simulink subsystem "PvtSubSys_VSM_LKA"  (R2020b)
settings: Solver=VariableStepAuto  StartTime=0.0  StopTime=10.0  RelTol=1e-3
values from neighbouring files (symbols this model uses):
  P_VSM_LKA_AbsEspInTime = 3.0    [LKA.sldd]
  P_VSM_LKA_absLongitudeAcceIn = 2.5    [LKA.sldd]
  P_VSM_LKA_absLongitudeAcceInTime = 3.0    [LKA.sldd]
  P_VSM_LKA_absLongitudeAcceOut = 3.0    [LKA.sldd]
  P_VSM_LKA_AccPedalPosnOut = 30.0    [LKA.sldd]
  P_VSM_LKA_AccPedalRateOutTime = 0.0    [LKA.sldd]
  P_VSM_LKA_AccRateIn = 30.0    [LKA.sldd]
  P_VSM_LKA_AccRateInTime = 1.5    [LKA.sldd]
  P_VSM_LKA_AccRateOut = 70.0    [LKA.sldd]
  P_VSM_LKA_BrakePressIn = 3.0    [LKA.sldd]
  P_VSM_LKA_BrakePressInTime = 1.5    [LKA.sldd]
  P_VSM_LKA_BrakePressOut = 5.0    [LKA.sldd]
  P_VSM_LKA_CurveFactor = 1.0    [LKA.sldd]
  P_VSM_LKA_DriverInputTrqValueIn = 2.0    [LKA.sldd]
  P_VSM_LKA_DriverInputTrqValueInTime = 3.0    [LKA.sldd]
  P_VSM_LKA_DriverInputTrqValueOut = 2.3    [LKA.sldd]
  P_VSM_LKA_EndSwitch = 1.0    [LKA.sldd]
  P_VSM_LKA_LaneChangeOffset = 0.11    [LKA.sldd]
  P_VSM_LKA_LaneCurveIn = 0.005    [LKA.sldd]
  P_VSM_LKA_LaneCurveOut = 0.006    [LKA.sldd]
  P_VSM_LKA_LateralAcceIn = 3.0    [LKA.sldd]
  P_VSM_LKA_LateralAcceInTime = 3.0    [LKA.sldd]
  P_VSM_LKA_LateralAcceOut = 3.5    [LKA.sldd]
  P_VSM_LKA_LongitudeAcceIn = 3.0    [LKA.sldd]
  P_VSM_LKA_LongitudeAcceOut = 3.5    [LKA.sldd]
  P_VSM_LKA_OverrideInTime = 1.5    [LKA.sldd]
  P_VSM_LKA_OverrideTime = 0.3    [LKA.sldd]
  P_VSM_LKA_OverrideValue = 1.2    [LKA.sldd]
  P_VSM_LKA_State_Absesp_enable = 1.0    [LKA.sldd]
  P_VSM_LKA_State_Accpedalrate_enable = 1.0    [LKA.sldd]
  P_VSM_LKA_State_Breakpressure_enable = 1.0    [LKA.sldd]
  P_VSM_LKA_State_DriverInputTrqValue_enable = 1.0    [LKA.sldd]
  P_VSM_LKA_State_Eps_enable = 1.0    [LKA.sldd]
  P_VSM_LKA_State_ESSSts_enable = 1.0    [LKA.sldd]
  P_VSM_LKA_State_Failsafe_enable = 1.0    [LKA.sldd]
  P_VSM_LKA_State_GEAR_enable = 1.0    [LKA.sldd]
  P_VSM_LKA_State_Handson_enable = 1.0    [LKA.sldd]
  P_VSM_LKA_State_Headingangle_enable = 1.0    [LKA.sldd]
  P_VSM_LKA_State_Lane_enable = 1.0    [LKA.sldd]
  P_VSM_LKA_State_LaneChange_enable = 1.0    [LKA.sldd]
  P_VSM_LKA_State_Lanecurve_enable = 1.0    [LKA.sldd]
  P_VSM_LKA_State_LateralAcce_enable = 1.0    [LKA.sldd]
  P_VSM_LKA_State_LongitudeAcc_enable = 1.0    [LKA.sldd]
  P_VSM_LKA_State_Overide_enable = 1.0    [LKA.sldd]
  P_VSM_LKA_State_Param_AngleOffset = 0.15    [LKA.sldd]
  P_VSM_LKA_State_Param_InterventionZoneIn = 0.4    [LKA.sldd]
  P_VSM_LKA_State_Param_InterventionZoneOut = -0.65    [LKA.sldd]
  P_VSM_LKA_State_Param_LaneCurve : value not decoded    [LKA.sldd]
  P_VSM_LKA_State_Param_LaneCurve_Offset : value not decoded    [LKA.sldd]
  P_VSM_LKA_State_Param_LaneWidth_Offset : value not decoded    [LKA.sldd]
  P_VSM_LKA_State_Param_OutOffset = 0.2    [LKA.sldd]
  P_VSM_LKA_State_Param_REInterventionZoneIn = 0.55    [LKA.sldd]
  P_VSM_LKA_State_Param_Sensitive_Offset : value not decoded    [LKA.sldd]
  P_VSM_LKA_State_SteerWheelAngle_enable = 1.0    [LKA.sldd]
  P_VSM_LKA_State_SteerWheelSpd_enable = 1.0    [LKA.sldd]
  P_VSM_LKA_State_TJASts_enable = 1.0    [LKA.sldd]
  P_VSM_LKA_State_TurnLight_enable = 1.0    [LKA.sldd]
  P_VSM_LKA_State_Vehspeed_enable = 1.0    [LKA.sldd]
  P_VSM_LKA_State_Yawsup_enable = 1.0    [LKA.sldd]
  P_VSM_LKA_SteerWheelAngleIn = 70.0    [LKA.sldd]
  P_VSM_LKA_SteerWheelAngleInTime = 3.0    [LKA.sldd]
  P_VSM_LKA_SteerWheelAngleOut = 90.0    [LKA.sldd]
  P_VSM_LKA_SteerWheelSpdIn = 150.0    [LKA.sldd]
  P_VSM_LKA_SteerWheelSpdInTime = 3.0    [LKA.sldd]
  P_VSM_LKA_SteerWheelSpdOut = 200.0    [LKA.sldd]
  P_VSM_LKA_TurnLightInTime = 3.0    [LKA.sldd]
  P_VSM_LKA_Warnarea1 = -0.55    [LKA.sldd]
  P_VSM_LKA_Warnarea2 = -0.35    [LKA.sldd]
  P_VSM_LKA_WarnInTime = 2.0    [LKA.sldd]
  P_VSM_LKA_WhelDy = 2.0    [LKA.sldd]
  P_VSM_LKA_YawRateIn = 0.2    [LKA.sldd]
  P_VSM_LKA_YawRateInTime = 1.0    [LKA.sldd]
  P_VSM_LKA_YawRateOut = 0.25    [LKA.sldd]
undefined symbols (not defined in the file or in its folder): P_VSM_LKA_AddOffset, P_VSM_LSMC_SampleTime, STATE
libraries: simulink x162
(part 2 of 5)

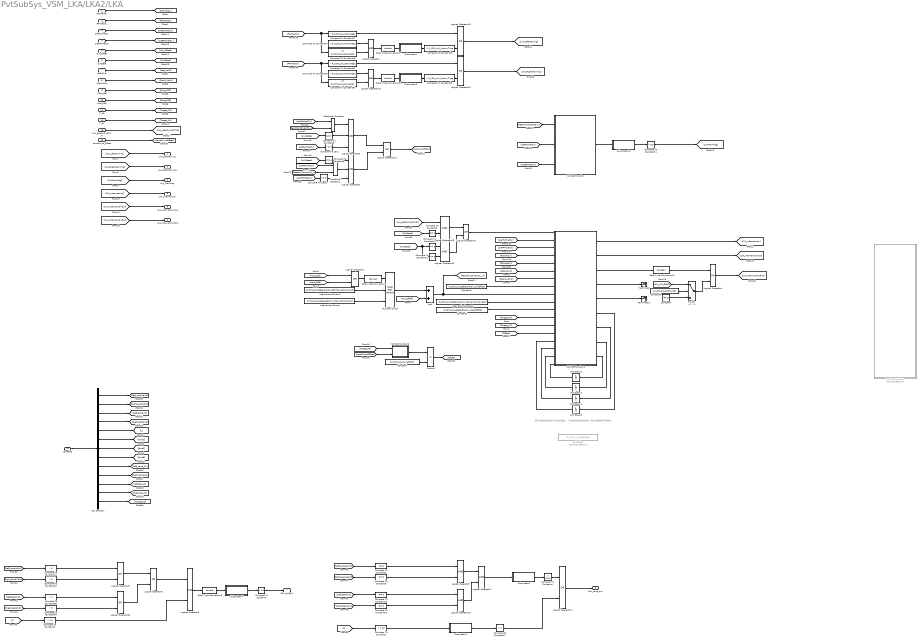
== system PvtSubSys_VSM_LKA/LKA2/LKA ==
  note: 基于车道线存在条件下成立的逻辑，一旦去掉车道线存在条件，那么该逻辑将不复存在；
  FLWhelDy : Inport
  FRWhelDy : Inport  Port=2
  preFLWhelDy : Inport  Port=3
  preFRWhelDy : Inport  Port=4
  LKA_Offset : Inport  Port=5
  LKAState : Inport  Port=6
  LeftValid : Inport  Port=7
  RightValid : Inport  Port=8
  Host_LRE : Inport  Port=9
  Host_RRE : Inport  Port=10
  T_A0 : Inport  Port=11
  T_A1 : Inport  Port=12
  LKA_READY2ACTIVE : Inport  Port=13
  LaneARe : Inport  Port=14
  LaneCurve_Offset : Inport  Port=15
  Add : Sum
  Bus Selector : BusSelector  OutputSignals=Left_LaneValid,Right_LaneValid,Left_ReValid,Right_ReValid,LDWLKAELK_LWidth,Signal_Lane1,Signal_Lane2,Signal_Lane3,Left_Lane_A1,Right_Lane_A1,Left_Re_A1,Right_Re_A1,T_A2
  Compare To Constant1 : simulink/Logic and Bit Operations/Compare To Constant  relop=<  const=2.45  OutDataTypeStr=boolean
  Compare To Constant10 : simulink/Logic and Bit Operations/Compare To Constant  relop=>=  const=3  OutDataTypeStr=boolean
  Compare To Constant11 : simulink/Logic and Bit Operations/Compare To Constant  relop=<=  const=5  OutDataTypeStr=boolean
  Compare To Constant12 : simulink/Logic and Bit Operations/Compare To Constant  relop=>  const=1  OutDataTypeStr=boolean
  Compare To Constant{3,6,13..14} (4 alike) : simulink/Logic and Bit Operations/Compare To Constant  relop===  const=0  OutDataTypeStr=boolean
  Compare To Constant{16,18,68,84} (4 alike) : simulink/Logic and Bit Operations/Compare To Constant  relop=>  const=0  OutDataTypeStr=boolean
  Compare To Constant2 : simulink/Logic and Bit Operations/Compare To Constant  relop=>  const=2.5  OutDataTypeStr=boolean
  Compare To Constant4 : simulink/Logic and Bit Operations/Compare To Constant  relop=>  const=0.25  OutDataTypeStr=boolean
  Compare To Constant44 : simulink/Logic and Bit Operations/Compare To Constant  relop=<  const=P_VSM_LKA_Warnarea2  OutDataTypeStr=boolean
  Compare To Constant45 : simulink/Logic and Bit Operations/Compare To Constant  relop=>  const=P_VSM_LKA_WarnInTime  OutDataTypeStr=boolean
  Compare To Constant46 : simulink/Logic and Bit Operations/Compare To Constant  relop=>=  const=P_VSM_LKA_Warnarea1  OutDataTypeStr=boolean
  Compare To Constant47 : simulink/Logic and Bit Operations/Compare To Constant  relop=<  const=P_VSM_LKA_Warnarea1  OutDataTypeStr=boolean
  Compare To Constant48 : simulink/Logic and Bit Operations/Compare To Constant  relop=<  const=P_VSM_LKA_Warnarea2  OutDataTypeStr=boolean
  Compare To Constant49 : simulink/Logic and Bit Operations/Compare To Constant  relop=>  const=P_VSM_LKA_WarnInTime  OutDataTypeStr=boolean
  Compare To Constant5 : simulink/Logic and Bit Operations/Compare To Constant  relop===  const=5  OutDataTypeStr=boolean
  Compare To Constant50 : simulink/Logic and Bit Operations/Compare To Constant  relop=>=  const=P_VSM_LKA_Warnarea1  OutDataTypeStr=boolean
  Compare To Constant51 : simulink/Logic and Bit Operations/Compare To Constant  relop=<  const=P_VSM_LKA_Warnarea1  OutDataTypeStr=boolean
  Compare To Constant7 : simulink/Logic and Bit Operations/Compare To Constant  relop=>  const=0.5  OutDataTypeStr=boolean
  Compare To Constant74 : simulink/Logic and Bit Operations/Compare To Constant  relop=>  const=0.5  OutDataTypeStr=boolean
  Compare To Constant8 : simulink/Logic and Bit Operations/Compare To Constant  relop===  const=4  OutDataTypeStr=boolean
  Compare To Constant9 : simulink/Logic and Bit Operations/Compare To Constant  relop===  const=2  OutDataTypeStr=boolean
  Compare To Zero : simulink/Logic and Bit Operations/Compare To Zero  relop=~=  OutDataTypeStr=boolean
  Compare To Zero1 : simulink/Logic and Bit Operations/Compare To Zero  relop=~=  OutDataTypeStr=boolean
  Constant : Constant  Value=P_VSM_LKA_CurveFactor
  Constant1 : Constant  Value=P_VSM_LKA_State_Param_OutOffset
  Constant2 : Constant  Value=P_VSM_LKA_State_Param_AngleOffset
  Constant3 : Constant  Value=P_VSM_LKA_EndSwitch
  Constant4 : Constant  Value=false  OutDataTypeStr=boolean
  Data Type Conversion : DataTypeConversion
  Data Type Conversion3 : DataTypeConversion  OutDataTypeStr=boolean
  Data Type Conversion5 : DataTypeConversion  OutDataTypeStr=double
  Data Type Conversion6 : DataTypeConversion  OutDataTypeStr=double
  Data Type Conversion8 : DataTypeConversion  OutDataTypeStr=double
  InterventionZoneIn : Constant  Value=P_VSM_LKA_State_Param_InterventionZoneIn
  InterventionZoneIn1 : Constant  Value=P_VSM_LKA_State_Param_REInterventionZoneIn
  InterventionZoneOut : Constant  Value=P_VSM_LKA_State_Param_InterventionZoneOut
  Logical Operator{,2,5,7,12..13,15,19} (8 alike) : Logic  AllPortsSameDT=off  OutDataTypeStr=boolean
  Logical Operator{1,3..4,6,10..11,14,18,20,26} (10 alike) : Logic  Operator=OR  AllPortsSameDT=off  OutDataTypeStr=boolean
  Logical Operator8 : Logic  Inputs=3  AllPortsSameDT=off  OutDataTypeStr=boolean
  Logical Operator9 : Logic  Inputs=3  AllPortsSameDT=off  OutDataTypeStr=boolean
  MATLAB Function : MATLAB Function  TreatAsAtomicUnit=on
  MATLAB Function1 : MATLAB Function  Commented=on  TreatAsAtomicUnit=on
  MATLAB Function2 : MATLAB Function  TreatAsAtomicUnit=on
  MATLAB Function3 : MATLAB Function  TreatAsAtomicUnit=on
  Multiport Switch : MultiPortSwitch  Inputs=2  DiagnosticForDefault=None
  Product : Product
  Relational Operator : RelationalOperator  Operator=<=  OutDataTypeStr=boolean  RndMeth=Simplest
  Relational Operator1 : RelationalOperator  Operator=<=  OutDataTypeStr=boolean  RndMeth=Simplest
  Subsystem1 : Subsystem  mask{Ts=P_VSM_LSMC_SampleTime, Max=10}
      mask prompts: Ts "Sample Time:"; Max "Max Limit:"
      mask Display:
      | Ts=get_param(gcb,'Ts');
      | Max=get_param(gcb,'Max');
      | disp(['Ts:' Ts '\n' 'Max:' Max ]);
  Subsystem10 : Subsystem  mask{Ts=P_VSM_LSMC_SampleTime, Max=10}
      mask prompts: Ts "Sample Time:"; Max "Max Limit:"
      mask Display:
      | Ts=get_param(gcb,'Ts');
      | Max=get_param(gcb,'Max');
      | disp(['Ts:' Ts '\n' 'Max:' Max ]);
  Subsystem2 : Subsystem  mask{Ts=P_VSM_LSMC_SampleTime, Max=10}
      mask prompts: Ts "Sample Time:"; Max "Max Limit:"
      mask Display:
      | Ts=get_param(gcb,'Ts');
      | Max=get_param(gcb,'Max');
      | disp(['Ts:' Ts '\n' 'Max:' Max ]);
  Subsystem3 : Subsystem  mask{Ts=P_VSM_LSMC_SampleTime, Max=10}
      mask prompts: Ts "Sample Time:"; Max "Max Limit:"
      mask Display:
      | Ts=get_param(gcb,'Ts');
      | Max=get_param(gcb,'Max');
      | disp(['Ts:' Ts '\n' 'Max:' Max ]);
  Subsystem4 : Subsystem  mask{Ts=P_VSM_LSMC_SampleTime, Max=10}
      mask prompts: Ts "Sample Time:"; Max "Max Limit:"
      mask Display:
      | Ts=get_param(gcb,'Ts');
      | Max=get_param(gcb,'Max');
      | disp(['Ts:' Ts '\n' 'Max:' Max ]);
  Subsystem7 : Subsystem  mask{Ts=P_VSM_LSMC_SampleTime, Max=10}
      mask prompts: Ts "Sample Time:"; Max "Max Limit:"
      mask Display:
      | Ts=get_param(gcb,'Ts');
      | Max=get_param(gcb,'Max');
      | disp(['Ts:' Ts '\n' 'Max:' Max ]);
  Switch : Switch  Criteria=u2 > Threshold
  Terminator : Terminator
  Terminator1 : Terminator
  Unit Delay{1..2,4..5} (4 alike) : UnitDelay  InitialCondition=single(0)  SampleTime=-1  HasFrameUpgradeWarning=on
  addOffset : Constant  Commented=on  Value=P_VSM_LKA_AddOffset
  LKA_LeftWarning : Outport
  LKA_RightWarning : Outport  Port=2
  LKA_Warnflag : Outport  Port=3
  LKA_Intervention : Outport  Port=4
  LKA_InterventionOut : Outport  Port=5
  LKA_InterventionEnd : Outport  Port=6
  ELK_Lane_in : Outport  Port=7
  ELK_Lane_out : Outport  Port=8
  wires:
  Constant4/1 -> Switch/3
  Constant3/1 -> Switch/2
  [VSM_LKA_END2] -> Switch/1
  Switch/1 -> Logical Operator4/2
  MATLAB Function3/5(rightactive) -> Terminator1/1  "VSM_LKA_rightactive"
  MATLAB Function3/4(leftactive) -> Terminator/1  "VSM_LKA_leftactive"
  Constant/1 -> Product/2
  Bus Selector/5 -> [L]  "<LDWLKAELK_LWidth>"
  Bus Selector/12 -> [Right_Re_A1]  "<Right_Re_A1>"
  Compare To Constant12/1 -> Logical Operator11/2
  [Right_LaneValid] -> Compare To Constant6/1
  Compare To Constant16/1 -> Logical Operator3/1
  Bus Selector/3 -> [Left_ReValid]  "<Left_ReValid>"
  Compare To Constant84/1 -> Logical Operator26/2
  Data Type Conversion8/1 -> Subsystem7/1(In1)
  Bus Selector/1 -> [Left_LaneValid]  "<Left_LaneValid>"
  Compare To Constant18/1 -> Logical Operator3/2
  Logical Operator26/1 -> Logical Operator6/2
  Compare To Constant3/1 -> Logical Operator7/1
  Bus Selector/9 -> [Left_Lane_A1]  "<Left_Lane_A1>"
  [L] -> Compare To Constant2/1
  [Left_LaneValid] -> Compare To Constant16/1
  Logical Operator6/1 -> Logical Operator5/1
  Bus Selector/2 -> [Right_LaneValid]  "<Right_LaneValid>"
  Subsystem4/1(Out1) -> Compare To Constant12/1
  [Right_ReValid] -> Compare To Constant14/1
  [Right_ReValid] -> Compare To Constant84/1
  Compare To Constant2/1 -> Logical Operator5/2
  [Left_ReValid] -> Compare To Constant13/1
  Compare To Constant68/1 -> Logical Operator26/1
  [Left_ReValid] -> Compare To Constant68/1
  Bus Selector/10 -> [Right_Lane_A1]  "<Right_Lane_A1>"
  Bus Selector/4 -> [Right_ReValid]  "<Right_ReValid>"
  Compare To Constant7/1 -> ELK_Lane_in/1
  [Left_LaneValid] -> Compare To Constant3/1
  Logical Operator15/1 -> Logical Operator2/2
  Compare To Constant4/1 -> Logical Operator11/1
  [L] -> Compare To Constant1/1
  Subsystem1/1(Out1) -> Compare To Constant4/1
  Compare To Constant1/1 -> Subsystem4/1(In1)
  Bus Selector/8 -> [lane3]  "<Signal_Lane3>"
  Bus Selector/7 -> [lane2]  "<Signal_Lane2>"
  Logical Operator11/1 -> ELK_Lane_out/1
  Compare To Constant13/1 -> Logical Operator15/1
  Subsystem7/1(Out1) -> Compare To Constant7/1
  Compare To Constant6/1 -> Logical Operator7/2
  [Right_LaneValid] -> Compare To Constant18/1
  Logical Operator2/1 -> Subsystem1/1(In1)
  Logical Operator3/1 -> Logical Operator6/1
  Bus Selector/11 -> [Left_Re_A1]  "<Left_Re_A1>"
  Compare To Constant14/1 -> Logical Operator15/2
  Logical Operator7/1 -> Logical Operator2/1
  LaneARe/1 -> Bus Selector/1
  Bus Selector/6 -> [lane1]  "<Signal_Lane1>"
  Logical Operator5/1 -> Data Type Conversion8/1
  [preFRWhelDy] -> MATLAB Function/3(preFRWhelDy)
  [preFLWhelDy] -> MATLAB Function/2(preFLWhelDy)
  Subsystem10/1(Out1) -> Compare To Constant74/1
  MATLAB Function/1(Warnflag) -> Subsystem10/1(In1)
  [ReactionZoneInDy_m] -> MATLAB Function/1(ReactionZoneInDy_m)
  Compare To Constant74/1 -> [LKAWarnflag]  "VSM_LKAWarnflag"
  MATLAB Function3/2(LKA_Out) -> [LKA_InterventionOut]  "VSM_LKA_LKAout"
  Compare To Constant10/1 -> Logical Operator12/1
  InterventionZoneIn1/1 -> Multiport Switch/2
  MATLAB Function3/1(LKA_active) -> [LKA_Intervention]  "VSM_LKA_LKAactive"
  Compare To Constant11/1 -> Logical Operator12/2
  InterventionZoneIn/1 -> Multiport Switch/3
  [preFRWhelDy] -> MATLAB Function3/3(PreFRWhelDy)
  [LKAState] -> Compare To Constant9/1
  [preFLWhelDy] -> MATLAB Function3/2(PreFLWhelDy)
  [Host_RRE] -> Logical Operator1/2
  MATLAB Function3/6(lfg) -> Unit Delay5/1
  [LKAState] -> Compare To Constant11/1, Compare To Constant10/1
  Unit Delay2/1 -> MATLAB Function3/18(routk1)
  Logical Operator12/1 -> Logical Operator14/2
  Compare To Constant9/1 -> Logical Operator13/2
  Unit Delay4/1 -> MATLAB Function3/16(loutk1)
  Unit Delay5/1 -> MATLAB Function3/15(lfgk1)
  MATLAB Function3/8(rfg) -> Unit Delay1/1
  [LKA_Offset] -> Add/2  "LKA_Offset"
  Multiport Switch/1 -> Add/1
  MATLAB Function3/7(lout) -> Unit Delay4/1
  MATLAB Function3/9(rout) -> Unit Delay2/1
  [LKA_READY2ACTIVE] -> Logical Operator13/1
  Constant1/1 -> MATLAB Function3/8(OutOffset)
  [FLWhelDy] -> MATLAB Function3/4(FLWhelDy)
  InterventionZoneOut/1 -> MATLAB Function3/10(ReactionZoneOutDy_m)
  [FRWhelDy] -> MATLAB Function3/5(FRWhelDy)
  [Target_A1] -> MATLAB Function3/13(HeadingAngel)
  Constant2/1 -> MATLAB Function3/11(Angleoffset)
  Unit Delay1/1 -> MATLAB Function3/17(rfgk1)
  Data Type Conversion/1 -> Multiport Switch/1
  Data Type Conversion3/1 -> Logical Operator4/1
  [Host_LRE] -> Logical Operator1/1
  MATLAB Function3/3(LKA_End) -> Data Type Conversion3/1
  [Left_Valid] -> MATLAB Function3/6(Left_Valid)
  Add/1 -> MATLAB Function3/9(ReactionZoneInDy_m), [ReactionZoneInDy_m]
  [Right_Valid] -> MATLAB Function3/7(Right_Valid)
  Logical Operator1/1 -> Data Type Conversion/1
  Logical Operator13/1 -> Logical Operator14/1
  Logical Operator4/1 -> [LKA_InterventionEnd]  "VSM_LKA_End"
  Logical Operator14/1 -> MATLAB Function3/1(active_fg)
  [Target_A0] -> MATLAB Function3/12(TargetLine)
  [preFRWhelDy] -> Compare To Zero1/1
  [preFLWhelDy] -> Relational Operator/1
  Compare To Zero/1 -> Logical Operator8/3
  [preFLWhelDy] -> Compare To Zero/1
  [ReactionZoneInDy_m] -> Relational Operator1/2
  Logical Operator9/1 -> Logical Operator10/2
  Logical Operator8/1 -> Logical Operator10/1
  Compare To Zero1/1 -> Logical Operator9/3
  [preFRWhelDy] -> Relational Operator1/1
  Logical Operator10/1 -> [VSM_LKA_END2]  "VSM_LKA_End2"
  Compare To Constant8/1 -> Logical Operator9/1
  [ReactionZoneInDy_m] -> Relational Operator/2
  Relational Operator/1 -> Logical Operator8/1
  Compare To Constant5/1 -> Logical Operator8/2
  [LKAState] -> Compare To Constant5/1
  Relational Operator1/1 -> Logical Operator9/2
  [LKAState] -> Compare To Constant8/1
  Compare To Constant45/1 -> Logical Operator18/2
  Subsystem3/1(Out1) -> Compare To Constant49/1
  Compare To Constant48/1 -> Logical Operator19/1
  Logical Operator/1 -> Data Type Conversion5/1
  Compare To Constant51/1 -> Logical Operator20/1
  Data Type Conversion6/1 -> Subsystem3/1(In1)
  Compare To Constant44/1 -> Logical Operator/1
  Compare To Constant46/1 -> Logical Operator/2
  Data Type Conversion5/1 -> Subsystem2/1(In1)
  Compare To Constant47/1 -> Logical Operator18/1
  Subsystem2/1(Out1) -> Compare To Constant45/1
  Compare To Constant49/1 -> Logical Operator20/2
  [FRWhelDy] -> Compare To Constant51/1, Compare To Constant48/1, Compare To Constant50/1
  Logical Operator18/1 -> [LKA_LeftWarning]  "VSM_LKA_LeftWarning"
  Compare To Constant50/1 -> Logical Operator19/2
  Logical Operator20/1 -> [LKA_RightWarning]  "VSM_LKA_RightWarning"
  [FLWhelDy] -> Compare To Constant47/1, Compare To Constant44/1, Compare To Constant46/1
  Logical Operator19/1 -> Data Type Conversion6/1
  LKA_READY2ACTIVE/1 -> [LKA_READY2ACTIVE]
  [LKA_InterventionEnd] -> LKA_InterventionEnd/1
  [LKA_InterventionOut] -> LKA_InterventionOut/1
  [LKA_Intervention] -> LKA_Intervention/1
  [LKAWarnflag] -> LKA_Warnflag/1
  [LKA_RightWarning] -> LKA_RightWarning/1
  [LKA_LeftWarning] -> LKA_LeftWarning/1
  LKAState/1 -> [LKAState]
  preFRWhelDy/1 -> [preFRWhelDy]
  preFLWhelDy/1 -> [preFLWhelDy]
  LKA_Offset/1 -> [LKA_Offset]
  T_A1/1 -> [Target_A1]
  T_A0/1 -> [Target_A0]
  LeftValid/1 -> [Left_Valid]
  RightValid/1 -> [Right_Valid]
  Host_RRE/1 -> [Host_RRE]
  Host_LRE/1 -> [Host_LRE]
  FRWhelDy/1 -> [FRWhelDy]
  FLWhelDy/1 -> [FLWhelDy]
  LaneCurve_Offset/1 -> [LaneCurveOffset]
  [LaneCurveOffset] -> MATLAB Function2/2(LaneCurveOffset)
  [Target_A2] -> MATLAB Function2/1(T_A2)
  Bus Selector/13 -> [Target_A2]  "<T_A2>"
  MATLAB Function2/1(Offset) -> Product/1
  Product/1 -> [Offset]
  [Offset] -> MATLAB Function3/14(LaneCurveOffset)
